simulink model "RSP"  (R2023a)
settings: Solver=FixedStepDiscrete  StartTime=0.0  StopTime=1.1*pri*N_observation  FixedStep=1.220703125E-8  RelTol=1e-3  EnableMultiTasking=on
model workspace (MAT data in the model file):
  Lambda : Simulink.Parameter (value not decoded)
  N_observation : Simulink.Parameter (value not decoded)
  N_sample : Simulink.Parameter (value not decoded)
  T_sampling : Simulink.Parameter (value not decoded)
  T_symbol : Simulink.Parameter (value not decoded)
  pri : Simulink.Parameter (value not decoded)
  symbol_delay : Simulink.Parameter (value not decoded)
symbols that are objects in the model workspace (value not decoded): Lambda, N_observation, N_sample, symbol_delay, T_sampling
libraries: hdlsllib x4, dsphdlxfrm2 x1
(part 11 of 49)

== matlab function RSP/Zero Signal ==
  data: y output
function y = fcn()
%#codegen

y = fi(zeros(8192 * 2,1),1,12);
